simulink model "Simulink_ZT_P4"  (R2021a)
settings: Solver=VariableStepAuto  StartTime=0.0  StopTime=5  RelTol=1e-3
values from neighbouring files (symbols this model uses):
  P4kTsch = P4kTschRnf * inv(P4TRnf)    [Praktikum.m]    (also in Praktikum_1.m = P4kTschRnf * P4TRnf)
  P4V = P4VKeinSprung    (= 0)    [Praktikum.m]    (also in Praktikum_1.m)
  P4VI = P4Vk(1)    [Praktikum.m]    (also in Praktikum_1.m)
  wsoll = 0.2    [Praktikum.m]    (also in Praktikum_1.m = 1)
  x0 = [0 0 0 0]    [Praktikum.m]    (also in Praktikum_1.m = [5 0 0 0])
  z0 = 0    [Praktikum.m]    (also in Praktikum_1.m)
  ZRM = ZRMGummi    [Praktikum.m]    (also in Praktikum_1.m; calcZRM.m = ss(A,bv,cT,d))
settings Model: Creator=janis  LastModifiedBy=janis

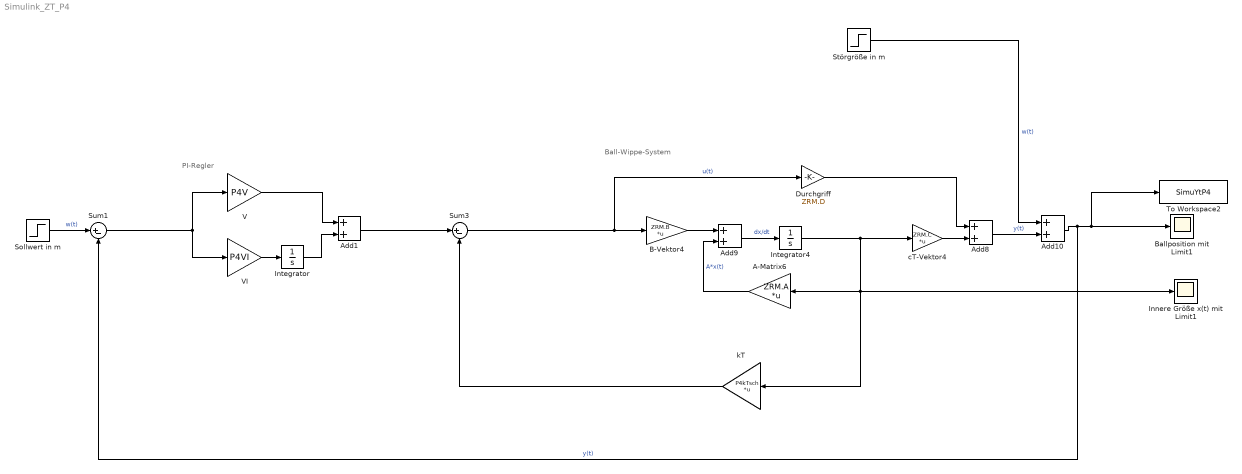
== system Simulink_ZT_P4 ==
  note: PI-Regler
  note: Ball-Wippe-System
  A-Matrix6 : Gain  Gain=ZRM.A  Multiplication=Matrix(K*u) (u vector)
  Add{1,8..10} (4 alike) : Sum
  B-Vektor4 : Gain  Gain=ZRM.B  Multiplication=Matrix(K*u) (u vector)
  Ballposition mit Limit1 : Scope
  Durchgriff : Gain  Gain=ZRM.D
  Innere Größe x(t) mit Limit1 : Scope
  Integrator : Integrator
  Integrator4 : Integrator  InitialCondition=x0
  Sollwert in m : Step  After=wsoll  SampleTime=0
  Störgröße in m : Step  Time=5  After=z0  SampleTime=0
  Sum1 : Sum  Inputs=|+-
  Sum3 : Sum  Inputs=|+-
  To Workspace2 : ToWorkspace  VariableName=SimuYtP4  SaveFormat=Timeseries  SampleTime=-1
  V : Gain  Gain=P4V
  VI : Gain  Gain=P4VI
  cT-Vektor4 : Gain  Gain=ZRM.C  Multiplication=Matrix(K*u) (u vector)
  kT : Gain  Gain=P4kTsch  Multiplication=Matrix(K*u) (u vector)
  wires:
  Add8/1 -> Add10/2  "y(t)"
  kT/1 -> Sum3/2
  A-Matrix6/1 -> Add9/2  "A*x(t)"
  Integrator4/1 -> cT-Vektor4/1, kT/1, A-Matrix6/1, Innere Größe x(t) mit Limit1/1
  Add10/1 -> Ballposition mit Limit1/1, To Workspace2/1, Sum1/2  "y(t)"
  cT-Vektor4/1 -> Add8/2
  Störgröße in m/1 -> Add10/1  "w(t)"
  B-Vektor4/1 -> Add9/1
  Sollwert in m/1 -> Sum1/1  "w(t)"
  Sum3/1 -> Durchgriff/1, B-Vektor4/1  "u(t)"
  Add9/1 -> Integrator4/1  "dx/dt"
  VI/1 -> Integrator/1
  V/1 -> Add1/1
  Sum1/1 -> VI/1, V/1
  Add1/1 -> Sum3/1
  Integrator/1 -> Add1/2
  Durchgriff/1 -> Add8/1
